simulink model "position_control_simulation_sm"  (R2023b)
settings: Solver=VariableStepAuto  StartTime=0.0  StopTime=10  RelTol=1e-12
undefined symbols (not defined in the file): A_t, B_t, K, Ts
settings Model: Creator=miche  LastModifiedBy=adamo

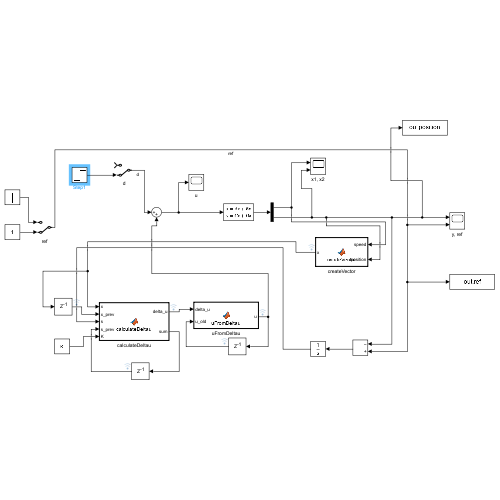
[thumbnail: Simulink's stored preview of the top-level diagram]
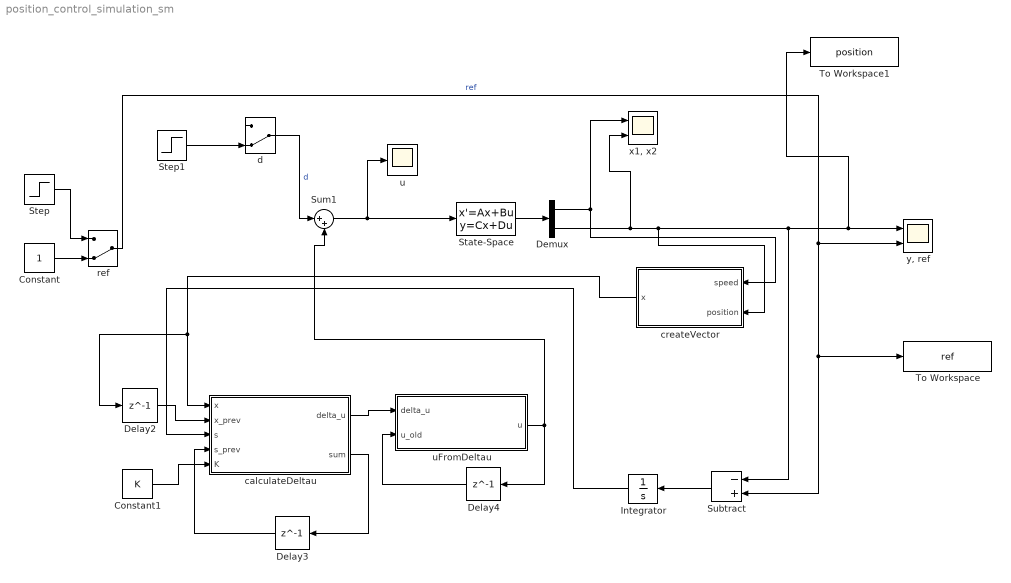
== system position_control_simulation_sm ==
  Constant : Constant
  Constant1 : Constant  Value=K
  Delay2 : Delay  DelayLength=1  InitialCondition=0  SampleTime=Ts
  Delay3 : Delay  DelayLength=1  InitialCondition=0  SampleTime=Ts
  Delay4 : Delay  DelayLength=1  InitialCondition=0  SampleTime=Ts
  Demux : Demux  Outputs=2
  Integrator : Integrator
  State-Space : StateSpace  A=A_t  B=B_t  C=eye(2)  D=[0; 0]  InitialCondition=[0,0]
  Step : Step  After=6.28  SampleTime=0
  Step1 : Step  Time=4  SampleTime=0
  Subtract : Sum  Inputs=-+
  Sum1 : Sum  Inputs=|++
  To Workspace : ToWorkspace  VariableName=ref  SaveFormat=Timeseries  SampleTime=-1
  To Workspace1 : ToWorkspace  VariableName=position  SaveFormat=Timeseries  SampleTime=-1
  calculateDeltau : MATLAB Function  TreatAsAtomicUnit=on
  createVector : MATLAB Function  TreatAsAtomicUnit=on
  d : ManualSwitch  CurrentSetting=0
  ref : ManualSwitch  CurrentSetting=0
  u : Scope
  uFromDeltau : MATLAB Function  TreatAsAtomicUnit=on
  "x1, x2" : Scope  NumInputPorts=2
  "y, ref" : Scope  NumInputPorts=2
  wires:
  Demux/1 -> createVector/1(speed), "x1, x2"/1
  State-Space/1 -> Demux/1
  Subtract/1 -> Integrator/1
  Step1/1 -> d/2
  ref/1 -> "y, ref"/2, To Workspace/1, Subtract/2  "ref"
  Step/1 -> ref/1
  Constant/1 -> ref/2
  Demux/2 -> createVector/2(position), Subtract/1, To Workspace1/1, "y, ref"/1, "x1, x2"/2
  d/1 -> Sum1/1  "d"
  Sum1/1 -> u/1, State-Space/1
  Delay3/1 -> calculateDeltau/4(s_prev)
  Integrator/1 -> calculateDeltau/3(s)
  calculateDeltau/1(delta_u) -> uFromDeltau/1(delta_u)
  Delay2/1 -> calculateDeltau/2(x_prev)
  Delay4/1 -> uFromDeltau/2(u_old)
  Constant1/1 -> calculateDeltau/5(K)
  uFromDeltau/1(u) -> Sum1/2, Delay4/1
  createVector/1(x) -> calculateDeltau/1(x), Delay2/1
  calculateDeltau/2(sum) -> Delay3/1

== matlab function position_control_simulation_sm/calculateDeltau ==
  data: x input; x_prev input; s input; s_prev input; K input; delta_u output; sum output
function [delta_u, sum]= calculateDeltau(x, x_prev, s, s_prev, K)
sum=s;

K1=K(1);
K2=K(2);
K_i=K(3);

delta_x = (x-x_prev);
delta_s = (s-s_prev);

a = -[K1 K2]* delta_x;

b = -K_i*delta_s;

delta_u = a+b;

== matlab function position_control_simulation_sm/uFromDeltau ==
  data: delta_u input; u_old input; u output
function u = uFromDeltau(delta_u, u_old)
    u = u_old+delta_u;
    if u < -12
        u=-12;
    end
    if u > 12
        u=12;
    end

== matlab function position_control_simulation_sm/createVector ==
  data: speed input; x output; position input
function x = createVector(speed,position)

x = [speed; position];
